simulink model "dvig"  (R2021b)
settings: Solver=ode14x  StartTime=0.0  StopTime=16  FixedStep=0.001  RelTol=1e-3
values from neighbouring files (symbols this model uses):
  F_s = 0.004    [init.m]
  Hu = 42.915e6    (= 42915000)    [init.m]
  I = 8.8e-4    (= 0.00088)    [init.m]
  i_g_arr = [377.41 480.99 586.62 694.69 805.34 918.56 1034.1 1151.8].*1000    [init.m]
  i_k_arr = [222.97 273.05 323.23 373.55 424.14 475.09 524.39 578.43].*1000    [init.m]
  K_arr = [0 1.48 2.96 4.44 5.92 7.40 8.88 10.36 11.84 13.32 14.80 22.20]    [init.m]
  k_tr_arr = [0.0174 0.087]    [init.m]
  k_v = 1.4    [init.m]
  kpd_gor = 0.98    [init.m]
  L0 = 14.627    [init.m]
  n_arr = [0 90457]    [init.m]
  R_arr = [510.7 463.9 424.2 390.9 363.4 341.2 323.5 310.9 301.3 294.0 289.6 288.2]    [init.m]
  R_v = 287    [init.m]
  sig_g = 0.955    [init.m]
  sig_s = 0.95    [init.m]
  sig_vh = 0.99    [init.m]
  T_g_arr = [373 473 573 673 773 873 973 1073]    [init.m]
  T_k_arr = [223.15 273.15 323.15 373.15 423.15 473.15 523.15 573.15]    [init.m]
  V_ks = F_ks*l_ks    (= 0.00176714586764)    [init.m]
undefined symbols (not defined in the file or in its folder): sigbuilder_block
libraries: aerolibatmos2 x1
settings Model: Creator=Admin  LastModifiedBy=admin
settings SolverCC: AlgebraicLoopSolver=TrustRegion
settings DataIOCC: ReturnWorkspaceOutputs=off
settings DebuggingCC: SFMachineParentedDataDiag=warning  ArithmeticOperatorsInVariantConditions=warning
settings SFSimCC: SimUseLocalCustomCode=off  CustomCodeUndefinedFunction=UseInterfaceOnly
settings RTWCC: RTWUseLocalCustomCode=off

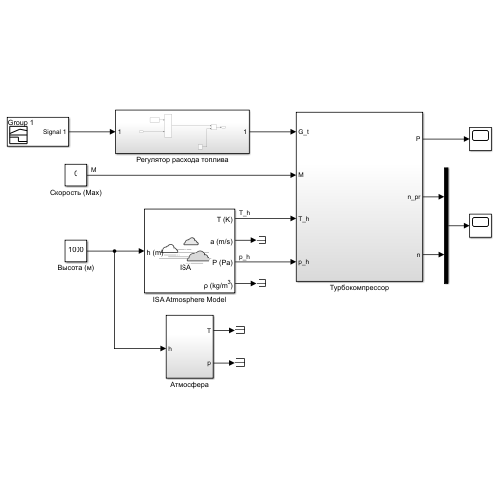
[thumbnail: Simulink's stored preview of the top-level diagram]
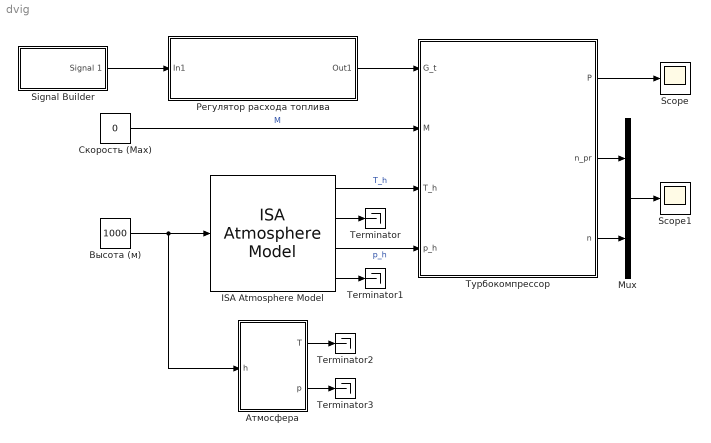
== system dvig ==
  ISA Atmosphere Model : aerolibatmos2/ISA Atmosphere Model  custom=off  g=9.80665  gamma=1.4  R=287.0531  L=0.0065  h_trop=11000  h_strat=20000  rho0=1.225  P0=101325  T0=288.15  h0=0
  Mux : Mux  Inputs=2
  Scope : Scope
  Scope1 : Scope
  Signal Builder : Subsystem  Tag=STV Subsys  LoadFcn=sigbuilder_block('load');  StartFcn=sigbuilder_block('start');  StopFcn=sigbuilder_block('stop');  ClipboardFcn=sigbuilder_block('clipboard');  mask(Sigbuilder block){tuvar=[0:10]}
      mask help: Simulink:masks:SigbuilderBlock_MD
      mask init:
      | if ~strcmp(get_param(bdroot(gcbh),'SimulationStatus'),'stopped') tuvar = sigbuilder_block('maskInit'); end
      settings: CopyFcn=sigbuilder_block('copy');  DeleteFcn=sigbuilder_block('delete');  ModelCloseFcn=sigbuilder_block('modelClose');  PreSaveFcn=sigbuilder_block('preSave');  PauseFcn=sigbuilder_block('pause');  ContinueFcn=sigbuilder_block('continue');  NameChangeFcn=sigbuilder_block('namechange');  OpenFcn=sigbuilder_block('open',[5.4 36 1141.2 516.6 ]);  CloseFcn=sigbuilder_block('close');
      mask Display: plot(0, 0, 100, 100,[2, 2, 32, 32, 2], [68, 8, 8, 68, 68],[32, 2], [38, 38], [32, 19, 2],[53, 60, 44], [32, 17, 17, 2],[16, 16, 31, 31]);txt = getActiveGroup(gcbh);text(2, 100, txt,'verticalAlignment', 'top');
  Terminator{,1..3} (4 alike) : Terminator
  Атмосфера : Subsystem
  Высота (м) : Constant  Value=1000
  Регулятор расхода топлива : Subsystem
  Скорость (Мах) : Constant  Value=0
  Турбокомпрессор : Subsystem
  wires:
  Высота (м)/1 -> Атмосфера/1(h), ISA Atmosphere Model/1
  ISA Atmosphere Model/4 -> Terminator1/1
  ISA Atmosphere Model/2 -> Terminator/1
  Скорость (Мах)/1 -> Турбокомпрессор/2(M)  "M"
  ISA Atmosphere Model/1 -> Турбокомпрессор/3(T_h)  "T_h"
  ISA Atmosphere Model/3 -> Турбокомпрессор/4(p_h)  "p_h"
  Турбокомпрессор/1(P) -> Scope/1
  Атмосфера/1(T) -> Terminator2/1
  Атмосфера/2(p) -> Terminator3/1
  Mux/1 -> Scope1/1
  Турбокомпрессор/3(n) -> Mux/2
  Турбокомпрессор/2(n_pr) -> Mux/1
  Signal Builder/1(Signal 1) -> Регулятор расхода топлива/1(In1)
  Регулятор расхода топлива/1(Out1) -> Турбокомпрессор/1(G_t)

== system dvig/Signal Builder ==
  Demux : Demux  Tag=STV Demux  Outputs=1
      settings: DisplayOption=none
  FromWs : FromWorkspace  Tag=STV FromWs  VariableName=tuvar
      SigBuilderData=|
      | common.afterFinalStr = 'Extrapolate'
      | common.sampleTime = 0
      | dataSet.timeRange = [0 16]
      | dataSet.name = 'Group 1'
      | sbobj.Groups.Name = 'Group 1'
      | sbobj.Groups.Signals.Name = 'Signal 1'
      | sbobj.Groups.Signals.XData = [0 1.06 3.8 5 6 8 10 12 14 16]
      | sbobj.Groups.Signals.YData = [0.001 0.00101 0.0023 0.0023 0.0051 0.0045 0.0078 0.0056 0.01225 0.01225]
      | sbobj.Groups.TimeRange = [0 16]
  Signal 1 : Outport  Tag=STV Outport
  wires:
  Demux/1 -> Signal 1/1
  FromWs/1 -> Demux/1

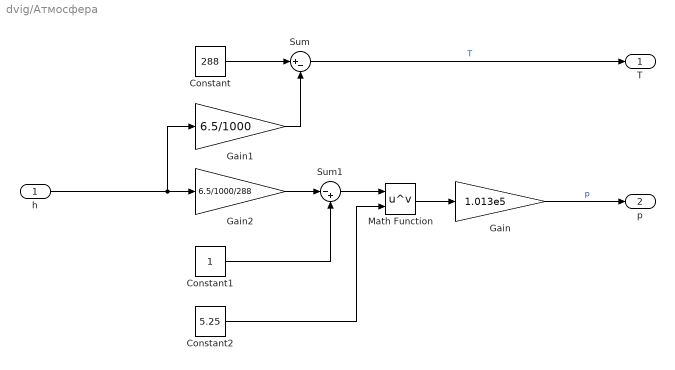
== system dvig/Атмосфера ==
  h : Inport
  Constant : Constant  Value=288
  Constant1 : Constant
  Constant2 : Constant  Value=5.25
  Gain : Gain  Gain=1.013e5
  Gain1 : Gain  Gain=6.5/1000
  Gain2 : Gain  Gain=6.5/1000/288
  Math Function : Math  Operator=pow  SaturateOnIntegerOverflow=on
  Sum : Sum  Inputs=|+-
  Sum1 : Sum  Inputs=|-+
  T : Outport  VectorParamsAs1DForOutWhenUnconnected=off
  p : Outport  Port=2  VectorParamsAs1DForOutWhenUnconnected=off
  wires:
  h/1 -> Gain1/1, Gain2/1
  Gain/1 -> p/1  "p"
  Sum1/1 -> Math Function/1
  Sum/1 -> T/1  "T"
  Constant1/1 -> Sum1/2
  Gain1/1 -> Sum/2
  Gain2/1 -> Sum1/1
  Constant2/1 -> Math Function/2
  Constant/1 -> Sum/1
  Math Function/1 -> Gain/1

== system dvig/Регулятор расхода топлива ==
  In1 : Inport
  Constant : Constant  Value=0.001
  Min : MinMax  Inputs=2
  Min1 : MinMax  Function=max  Inputs=2
  n_max : Constant  Value=0.0084
  Out1 : Outport
  wires:
  Min/1 -> Min1/1
  n_max/1 -> Min/1
  Constant/1 -> Min1/2
  Min1/1 -> Out1/1
  In1/1 -> Min/2

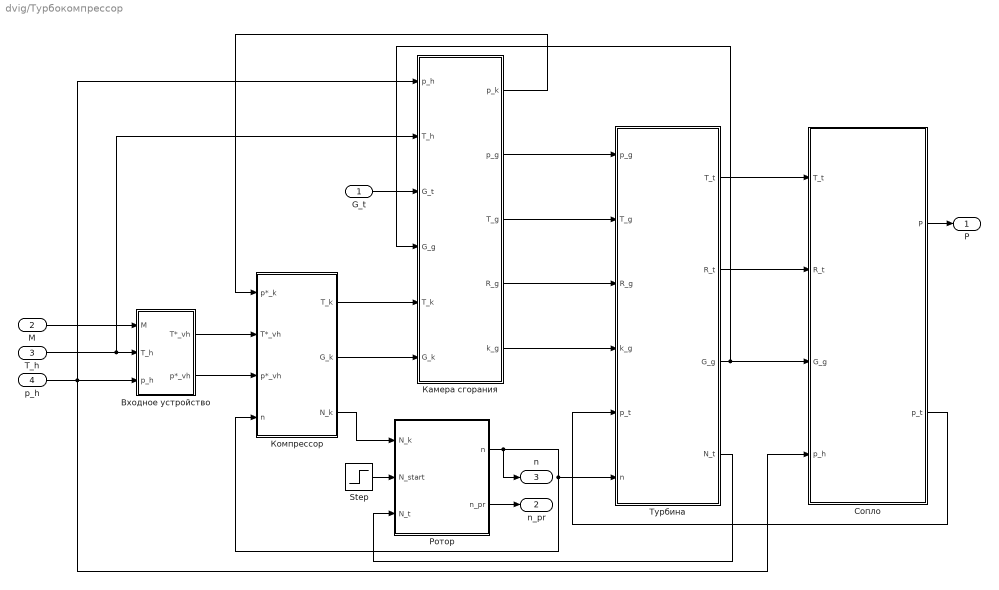
== system dvig/Турбокомпрессор ==
  G_t : Inport
  M : Inport  Port=2
  T_h : Inport  Port=3
  p_h : Inport  Port=4
  Step : Step  Time=3  Before=60000  After=0  SampleTime=0
  Входное устройство : Subsystem
  Камера сгорания : Subsystem
  Компрессор : Subsystem
  Ротор : Subsystem
  Сопло : Subsystem
  Турбина : Subsystem
  P : Outport  VectorParamsAs1DForOutWhenUnconnected=off
  n_pr : Outport  Port=2  VectorParamsAs1DForOutWhenUnconnected=off
  n : Outport  Port=3  VectorParamsAs1DForOutWhenUnconnected=off
  wires:
  G_t/1 -> Камера сгорания/3(G_t)
  Камера сгорания/1(p_k) -> Компрессор/1(p*_k)
  Входное устройство/1(T*_vh) -> Компрессор/2(T*_vh)
  Компрессор/1(T_k) -> Камера сгорания/5(T_k)
  T_h/1 -> Камера сгорания/2(T_h), Входное устройство/2(T_h)
  p_h/1 -> Камера сгорания/1(p_h), Входное устройство/3(p_h), Сопло/4(p_h)
  M/1 -> Входное устройство/1(M)
  Компрессор/2(G_k) -> Камера сгорания/6(G_k)
  Входное устройство/2(p*_vh) -> Компрессор/3(p*_vh)
  Камера сгорания/3(T_g) -> Турбина/2(T_g)
  Камера сгорания/4(R_g) -> Турбина/3(R_g)
  Камера сгорания/5(k_g) -> Турбина/4(k_g)
  Камера сгорания/2(p_g) -> Турбина/1(p_g)
  Ротор/1(n) -> n/1, Турбина/6(n), Компрессор/4(n)
  Сопло/2(p_t) -> Турбина/5(p_t)
  Компрессор/3(N_k) -> Ротор/1(N_k)
  Турбина/1(T_t) -> Сопло/1(T_t)
  Турбина/2(R_t) -> Сопло/2(R_t)
  Сопло/1(P) -> P/1
  Турбина/4(N_t) -> Ротор/3(N_t)
  Step/1 -> Ротор/2(N_start)
  Турбина/3(G_g) -> Сопло/3(G_g), Камера сгорания/4(G_g)
  Ротор/2(n_pr) -> n_pr/1

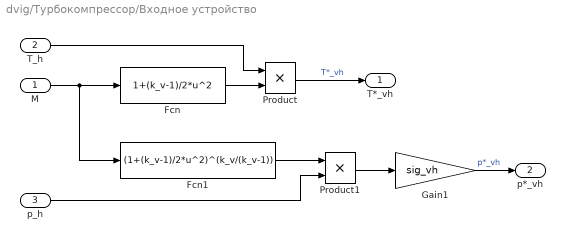
== system dvig/Турбокомпрессор/Входное устройство ==
  M : Inport
  T_h : Inport  Port=2
  p_h : Inport  Port=3
  Fcn : Fcn  Expr=1+(k_v-1)/2*u^2
  Fcn1 : Fcn  Expr=(1+(k_v-1)/2*u^2)^(k_v/(k_v-1))
  Gain1 : Gain  Gain=sig_vh
  Product : Product
  Product1 : Product
  T*_vh : Outport  VectorParamsAs1DForOutWhenUnconnected=off
  p*_vh : Outport  Port=2  VectorParamsAs1DForOutWhenUnconnected=off
  wires:
  p_h/1 -> Product1/2
  T_h/1 -> Product/1
  Product/1 -> T*_vh/1  "T*_vh"
  Fcn1/1 -> Product1/1
  Fcn/1 -> Product/2
  Gain1/1 -> p*_vh/1  "p*_vh"
  M/1 -> Fcn1/1, Fcn/1
  Product1/1 -> Gain1/1

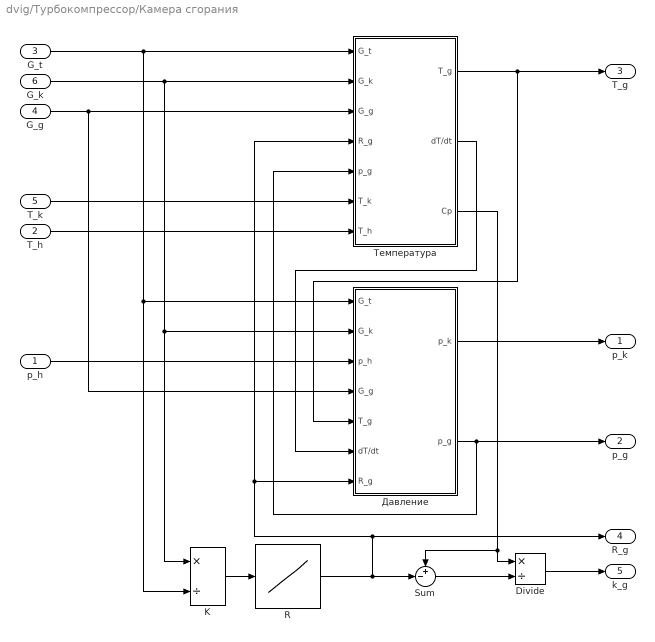
== system dvig/Турбокомпрессор/Камера сгорания ==
  p_h : Inport
  T_h : Inport  Port=2
  G_t : Inport  Port=3
  G_g : Inport  Port=4
  T_k : Inport  Port=5
  G_k : Inport  Port=6
  Divide : Product  Inputs=*/
  K : Product  Inputs=*/
  R : Lookup_n-D  NumberOfTableDimensions=1  BreakpointsForDimension1=K_arr  Table=R_arr  InternalRulePriority=Speed  RndMeth=Simplest  InputSameDT=on
  Sum : Sum  Inputs=+-|
  Давление : Subsystem
  Температура : Subsystem
  p_k : Outport  VectorParamsAs1DForOutWhenUnconnected=off
  p_g : Outport  Port=2  VectorParamsAs1DForOutWhenUnconnected=off
  T_g : Outport  Port=3  VectorParamsAs1DForOutWhenUnconnected=off
  R_g : Outport  Port=4  VectorParamsAs1DForOutWhenUnconnected=off
  k_g : Outport  Port=5  VectorParamsAs1DForOutWhenUnconnected=off
  wires:
  G_t/1 -> K/2, Давление/1(G_t), Температура/1(G_t)
  G_k/1 -> K/1, Давление/2(G_k), Температура/2(G_k)
  p_h/1 -> Давление/3(p_h)
  G_g/1 -> Давление/4(G_g), Температура/3(G_g)
  K/1 -> R/1
  R/1 -> R_g/1, Температура/4(R_g), Давление/7(R_g), Sum/2
  Sum/1 -> Divide/2
  Температура/3(Cp) -> Divide/1, Sum/1
  Давление/1(p_k) -> p_k/1
  Давление/2(p_g) -> Температура/5(p_g), p_g/1
  Температура/1(T_g) -> Давление/5(T_g), T_g/1
  Температура/2(dT/dt) -> Давление/6(dT/dt)
  T_k/1 -> Температура/6(T_k)
  T_h/1 -> Температура/7(T_h)
  Divide/1 -> k_g/1

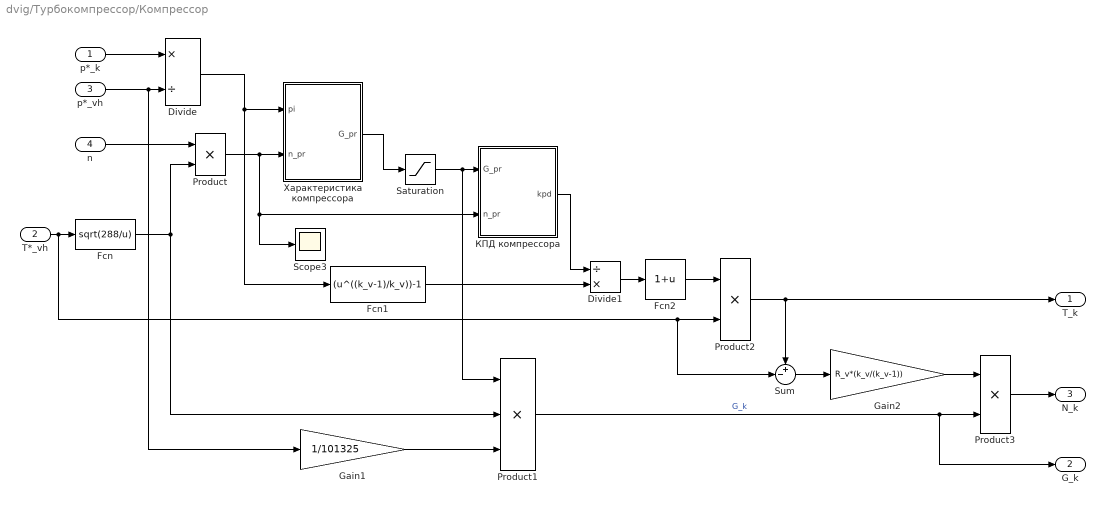
== system dvig/Турбокомпрессор/Компрессор ==
  p*_k : Inport
  T*_vh : Inport  Port=2
  p*_vh : Inport  Port=3
  n : Inport  Port=4
  Divide : Product  Inputs=*/
  Divide1 : Product  Inputs=/*
  Fcn : Fcn  Expr=sqrt(288/u)
  Fcn1 : Fcn  Expr=(u^((k_v-1)/k_v))-1
  Fcn2 : Fcn  Expr=1+u
  Gain1 : Gain  Gain=1/101325
  Gain2 : Gain  Gain=R_v*(k_v/(k_v-1))
  Product : Product
  Product1 : Product  Inputs=3
  Product2 : Product
  Product3 : Product
  Saturation : Saturate  UpperLimit=0.8  LowerLimit=0.05
  Scope3 : Scope
  Sum : Sum  Inputs=+-|
  КПД компрессора : MATLAB Function  TreatAsAtomicUnit=on
  Характеристика компрессора : MATLAB Function  TreatAsAtomicUnit=on
  T_k : Outport  VectorParamsAs1DForOutWhenUnconnected=off
  G_k : Outport  Port=2  VectorParamsAs1DForOutWhenUnconnected=off
  N_k : Outport  Port=3  VectorParamsAs1DForOutWhenUnconnected=off
  wires:
  p*_k/1 -> Divide/1
  Divide/1 -> Fcn1/1, Характеристика компрессора/1(pi)
  Saturation/1 -> Product1/1, КПД компрессора/1(G_pr)
  p*_vh/1 -> Gain1/1, Divide/2
  Fcn2/1 -> Product2/1
  Gain1/1 -> Product1/3
  Fcn/1 -> Product1/2, Product/2
  Divide1/1 -> Fcn2/1
  Sum/1 -> Gain2/1
  Product/1 -> Scope3/1, КПД компрессора/2(n_pr), Характеристика компрессора/2(n_pr)
  n/1 -> Product/1
  Gain2/1 -> Product3/1
  Product1/1 -> G_k/1, Product3/2  "G_k"
  Product3/1 -> N_k/1
  T*_vh/1 -> Sum/2, Product2/2, Fcn/1
  КПД компрессора/1(kpd) -> Divide1/1
  Product2/1 -> T_k/1, Sum/1
  Fcn1/1 -> Divide1/2
  Характеристика компрессора/1(G_pr) -> Saturation/1

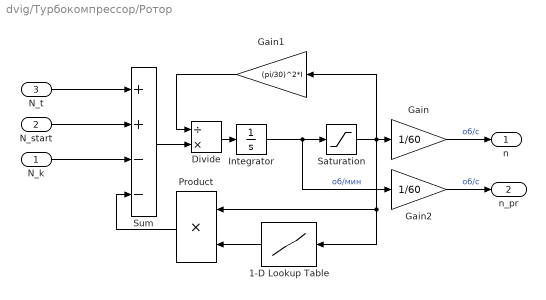
== system dvig/Турбокомпрессор/Ротор ==
  N_k : Inport
  N_start : Inport  Port=2
  N_t : Inport  Port=3
  1-D Lookup Table : Lookup_n-D  NumberOfTableDimensions=1  BreakpointsForDimension1=n_arr  Table=k_tr_arr  InternalRulePriority=Speed  RndMeth=Simplest  InputSameDT=on
  Divide : Product  Inputs=/*
  Gain : Gain  Gain=1/60
  Gain1 : Gain  Gain=(pi/30)^2*I
  Gain2 : Gain  Gain=1/60
  Integrator : Integrator
  Product : Product
  Saturation : Saturate  UpperLimit=90500  LowerLimit=1
  Sum : Sum  Inputs=++--
  n : Outport  VectorParamsAs1DForOutWhenUnconnected=off
  n_pr : Outport  Port=2  VectorParamsAs1DForOutWhenUnconnected=off
  wires:
  N_k/1 -> Sum/3
  N_t/1 -> Sum/1
  Saturation/1 -> 1-D Lookup Table/1, Product/1, Gain/1, Gain1/1
  Integrator/1 -> Gain2/1, Saturation/1  "об/мин"
  Gain/1 -> n/1  "об/с"
  Sum/1 -> Divide/2
  Divide/1 -> Integrator/1
  Gain1/1 -> Divide/1
  1-D Lookup Table/1 -> Product/2
  Product/1 -> Sum/4
  N_start/1 -> Sum/2
  Gain2/1 -> n_pr/1  "об/с"

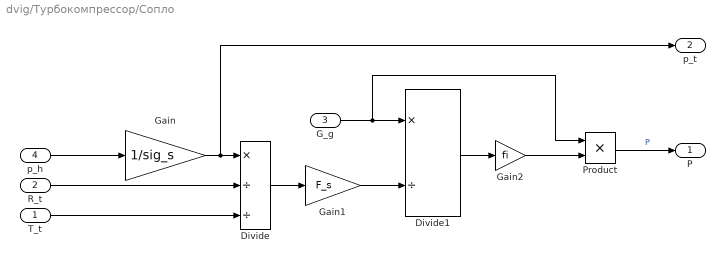
== system dvig/Турбокомпрессор/Сопло ==
  T_t : Inport
  R_t : Inport  Port=2
  G_g : Inport  Port=3
  p_h : Inport  Port=4
  Divide : Product  Inputs=*//
  Divide1 : Product  Inputs=*/
  Gain : Gain  Gain=1/sig_s
  Gain1 : Gain  Gain=F_s
  Gain2 : Gain  Gain=fi
  Product : Product
  P : Outport  VectorParamsAs1DForOutWhenUnconnected=off
  p_t : Outport  Port=2  VectorParamsAs1DForOutWhenUnconnected=off
  wires:
  T_t/1 -> Divide/3
  p_h/1 -> Gain/1
  R_t/1 -> Divide/2
  Divide1/1 -> Gain2/1
  G_g/1 -> Product/1, Divide1/1
  Product/1 -> P/1  "P"
  Divide/1 -> Gain1/1
  Gain2/1 -> Product/2
  Gain/1 -> p_t/1, Divide/1
  Gain1/1 -> Divide1/2

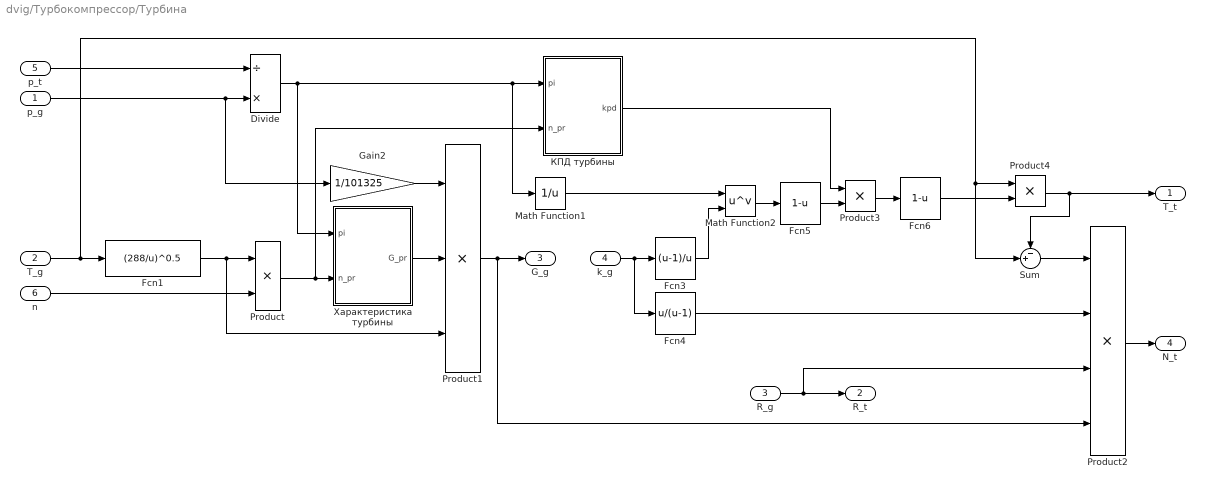
== system dvig/Турбокомпрессор/Турбина ==
  p_g : Inport
  T_g : Inport  Port=2
  R_g : Inport  Port=3
  k_g : Inport  Port=4
  p_t : Inport  Port=5
  n : Inport  Port=6
  Divide : Product  Inputs=/*
  Fcn1 : Fcn  Expr=(288/u)^0.5
  Fcn3 : Fcn  Expr=(u-1)/u
  Fcn4 : Fcn  Expr=u/(u-1)
  Fcn5 : Fcn  Expr=1-u
  Fcn6 : Fcn  Expr=1-u
  Gain2 : Gain  Gain=1/101325
  Math Function1 : Math  Operator=reciprocal  SignedPower=on  SaturateOnIntegerOverflow=on
  Math Function2 : Math  Operator=pow  SaturateOnIntegerOverflow=on
  Product : Product
  Product1 : Product  Inputs=3
  Product2 : Product  Inputs=4
  Product3 : Product
  Product4 : Product
  Sum : Sum  Inputs=-+|
  КПД турбины : MATLAB Function  TreatAsAtomicUnit=on
  Характеристика турбины : MATLAB Function  TreatAsAtomicUnit=on
  T_t : Outport  VectorParamsAs1DForOutWhenUnconnected=off
  R_t : Outport  Port=2  VectorParamsAs1DForOutWhenUnconnected=off
  G_g : Outport  Port=3  VectorParamsAs1DForOutWhenUnconnected=off
  N_t : Outport  Port=4  VectorParamsAs1DForOutWhenUnconnected=off
  wires:
  n/1 -> Product/2
  p_t/1 -> Divide/1
  p_g/1 -> Gain2/1, Divide/2
  Divide/1 -> Math Function1/1, КПД турбины/1(pi), Характеристика турбины/1(pi)
  Fcn1/1 -> Product1/3, Product/1
  R_g/1 -> Product2/3, R_t/1
  Product/1 -> КПД турбины/2(n_pr), Характеристика турбины/2(n_pr)
  Product1/1 -> G_g/1, Product2/4
  Fcn3/1 -> Math Function2/2
  k_g/1 -> Fcn4/1, Fcn3/1
  Fcn4/1 -> Product2/2
  Math Function2/1 -> Fcn5/1
  Fcn5/1 -> Product3/2
  Product3/1 -> Fcn6/1
  Product2/1 -> N_t/1
  Fcn6/1 -> Product4/2
  Product4/1 -> Sum/1, T_t/1
  Sum/1 -> Product2/1
  T_g/1 -> Sum/2, Product4/1, Fcn1/1
  Math Function1/1 -> Math Function2/1
  Характеристика турбины/1(G_pr) -> Product1/2
  КПД турбины/1(kpd) -> Product3/1
  Gain2/1 -> Product1/1

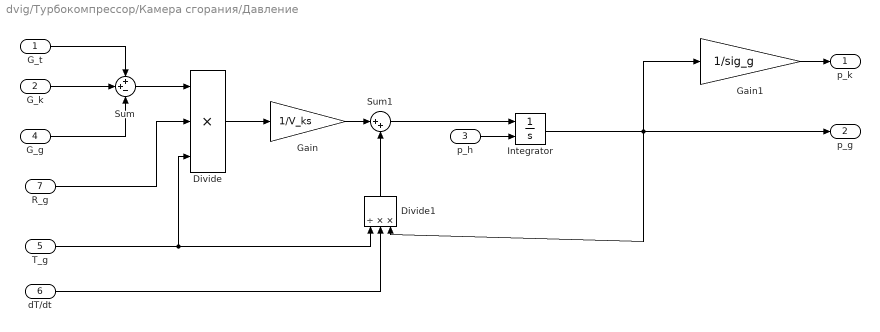
== system dvig/Турбокомпрессор/Камера сгорания/Давление ==
  G_t : Inport
  G_k : Inport  Port=2
  p_h : Inport  Port=3
  G_g : Inport  Port=4
  T_g : Inport  Port=5
  dT/dt : Inport  Port=6
  R_g : Inport  Port=7
  Divide : Product  Inputs=3
  Divide1 : Product  Inputs=/**
  Gain : Gain  Gain=1/V_ks
  Gain1 : Gain  Gain=1/sig_g
  Integrator : Integrator  InitialConditionSource=external
  Sum : Sum  Inputs=++-
  Sum1 : Sum  Inputs=|++
  p_k : Outport  VectorParamsAs1DForOutWhenUnconnected=off
  p_g : Outport  Port=2  VectorParamsAs1DForOutWhenUnconnected=off
  wires:
  Gain1/1 -> p_k/1
  Integrator/1 -> Divide1/3, p_g/1, Gain1/1
  G_g/1 -> Sum/3
  G_k/1 -> Sum/2
  G_t/1 -> Sum/1
  Gain/1 -> Sum1/1
  Divide/1 -> Gain/1
  Sum/1 -> Divide/1
  T_g/1 -> Divide1/1, Divide/3
  p_h/1 -> Integrator/2
  Divide1/1 -> Sum1/2
  Sum1/1 -> Integrator/1
  dT/dt/1 -> Divide1/2
  R_g/1 -> Divide/2

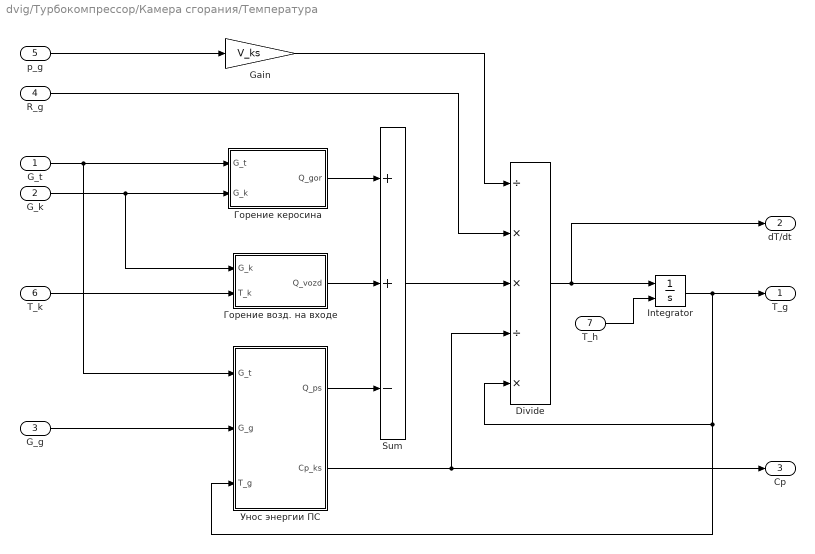
== system dvig/Турбокомпрессор/Камера сгорания/Температура ==
  G_t : Inport
  G_k : Inport  Port=2
  G_g : Inport  Port=3
  R_g : Inport  Port=4
  p_g : Inport  Port=5
  T_k : Inport  Port=6
  T_h : Inport  Port=7
  Divide : Product  Inputs=/**/*
  Gain : Gain  Gain=V_ks
  Integrator : Integrator  InitialConditionSource=external
  Sum : Sum  Inputs=++-
  Горение возд. на входе : Subsystem
  Горение керосина : Subsystem
  Унос энергии ПС : Subsystem
  T_g : Outport  VectorParamsAs1DForOutWhenUnconnected=off
  dT/dt : Outport  Port=2  VectorParamsAs1DForOutWhenUnconnected=off
  Cp : Outport  Port=3  VectorParamsAs1DForOutWhenUnconnected=off
  wires:
  G_t/1 -> Унос энергии ПС/1(G_t), Горение керосина/1(G_t)
  G_k/1 -> Горение возд. на входе/1(G_k), Горение керосина/2(G_k)
  Горение керосина/1(Q_gor) -> Sum/1
  Sum/1 -> Divide/3
  R_g/1 -> Divide/2
  p_g/1 -> Gain/1
  Gain/1 -> Divide/1
  T_h/1 -> Integrator/2
  Divide/1 -> Integrator/1, dT/dt/1
  Integrator/1 -> T_g/1, Унос энергии ПС/3(T_g), Divide/5
  T_k/1 -> Горение возд. на входе/2(T_k)
  Горение возд. на входе/1(Q_vozd) -> Sum/2
  G_g/1 -> Унос энергии ПС/2(G_g)
  Унос энергии ПС/1(Q_ps) -> Sum/3
  Унос энергии ПС/2(Cp_ks) -> Cp/1, Divide/4

== system dvig/Турбокомпрессор/Камера сгорания/Температура/Горение возд. на входе ==
  G_k : Inport
  T_k : Inport  Port=2
  Divide1 : Product  Inputs=*/
  Product : Product  Inputs=3
  i_k : Lookup_n-D  NumberOfTableDimensions=1  BreakpointsForDimension1=T_k_arr  Table=i_k_arr  InternalRulePriority=Speed  RndMeth=Simplest  InputSameDT=on
  Q_vozd : Outport  VectorParamsAs1DForOutWhenUnconnected=off
  wires:
  Product/1 -> Q_vozd/1
  G_k/1 -> Product/1
  Divide1/1 -> Product/2
  i_k/1 -> Divide1/1
  T_k/1 -> Divide1/2, Product/3, i_k/1

== system dvig/Турбокомпрессор/Камера сгорания/Температура/Горение керосина ==
  G_t : Inport
  G_k : Inport  Port=2
  Gain : Gain  Gain=1/L0
  Gain1 : Gain  Gain=Hu*kpd_gor
  MinMax : MinMax  Inputs=2
  Q_gor : Outport  VectorParamsAs1DForOutWhenUnconnected=off
  wires:
  MinMax/1 -> Gain1/1
  G_t/1 -> MinMax/1
  G_k/1 -> Gain/1
  Gain1/1 -> Q_gor/1  "Q_gor"
  Gain/1 -> MinMax/2

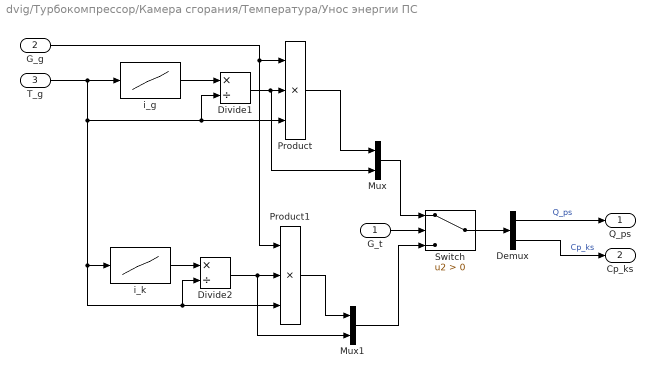
== system dvig/Турбокомпрессор/Камера сгорания/Температура/Унос энергии ПС ==
  G_t : Inport
  G_g : Inport  Port=2
  T_g : Inport  Port=3
  Demux : Demux  Outputs=2
  Divide1 : Product  Inputs=*/
  Divide2 : Product  Inputs=*/
  Mux : Mux  Inputs=2
  Mux1 : Mux  Inputs=2
  Product : Product  Inputs=3
  Product1 : Product  Inputs=3
  Switch : Switch  Criteria=u2 > Threshold
  i_g : Lookup_n-D  NumberOfTableDimensions=1  BreakpointsForDimension1=T_g_arr  Table=i_g_arr  InternalRulePriority=Speed  RndMeth=Simplest  InputSameDT=on
  i_k : Lookup_n-D  NumberOfTableDimensions=1  BreakpointsForDimension1=T_k_arr  Table=i_k_arr  InternalRulePriority=Speed  RndMeth=Simplest  InputSameDT=on
  Q_ps : Outport  VectorParamsAs1DForOutWhenUnconnected=off
  Cp_ks : Outport  Port=2  VectorParamsAs1DForOutWhenUnconnected=off
  wires:
  Divide2/1 -> Mux1/2, Product1/2
  G_t/1 -> Switch/2
  Demux/2 -> Cp_ks/1  "Cp_ks"
  Mux1/1 -> Switch/3
  i_k/1 -> Divide2/1
  Product1/1 -> Mux1/1
  Mux/1 -> Switch/1
  i_g/1 -> Divide1/1
  Demux/1 -> Q_ps/1  "Q_ps"
  Switch/1 -> Demux/1
  Divide1/1 -> Mux/2, Product/2
  G_g/1 -> Product1/1, Product/1
  Product/1 -> Mux/1
  T_g/1 -> Divide2/2, Product1/3, i_k/1, Divide1/2, Product/3, i_g/1

== matlab function dvig/Турбокомпрессор/Турбина/Характеристика турбины ==
  data: pi input; n_pr input; G_pr output
%function G_pr = inter(pi,n_pr)
function G_pr = inter(pi, n_pr)
    mas = [0 381.82 534.53 686.8 763.6 836.5 ...
    1 1.0000 1.0000 1.0000 1.0000 1.0000 ...
    1 1.2000 1.2000 1.2000 1.2000 1.2000 ...
    1 1.5500 1.5328 1.5321 1.5316 1.5327 ...
    1 1.7000 1.7300 1.7418 1.7413 1.7409 ...
    1 2.0216 2.0172 2.0170 2.0169 2.0168 ...
    1 3.4511 3.4473 3.4496 3.4509 3.4509 ...
    1 4.7626 4.7530 4.7589 4.7605 4.8437 ...
    1 6.1721 6.2159 6.3032 6.3527 6.3440 ...
    0 0.000000 0.000000 0.000000 0.000000 0.000000 ...
    0 0.220000 0.225000 0.220000 0.215000 0.216000 ...
    0 0.292801 0.296743 0.297500 0.297700 0.298700 ...
    0 0.303760 0.306989 0.309100 0.309585 0.310585 ...
    0 0.311119 0.315387 0.316097 0.316300 0.317300 ...
    0 0.318322 0.320272 0.320966 0.321209 0.322209 ...
    0 0.318560 0.320411 0.321058 0.321212 0.322212 ...
    0 0.318617 0.320429 0.321185 0.321266 0.322266];

    M = 16;
    N = 6;

    N1 = M/2;
    Gkpd = zeros(1,M);
    k1 = 0;
    k2 = 0;
    XA = 0;
    XB = 0;
    kpd = 0;
    
    %
    G_pr = 0;
    %
    if n_pr>mas(N)
        kp=1+N-2;
        ks=1+N-1;
        XA=mas(kp);
        XB=mas(ks);
        k1=1-2+N*2;
        k2=1-1+N*2;

        for i=1:1:M
            kq=k1+(i-1)*N;
            kw=k2+(i-1)*N;
            if XB==XA
                XB=XB+0.1;
            end

            Gkpd(i)=mas(kq)+(((mas(kw)-mas(kq))*(n_pr-XA))/(XB-XA));
        end

    end
    
    if n_pr<mas(1)
        XA=mas(1);
        XB=mas(2);
        k1=N+1;
        k2=N+2;
        for i=1:1:M
            kq=k1+(i-1)*N;
            kw=k2+(i-1)*N;
            if XB==XA
                XB=XB+0.1;
            end
    
            Gkpd(i)=mas(kq)+(((mas(kw)-mas(kq))*(n_pr-XA))/(XB-XA));
        end
    
    else
        for i=1:1:N-1
            if n_pr>=mas(i)
                if n_pr<=mas(i+1)
                    XA=mas(i);
                    XB=mas(i+1);
                    k1=N+i;
                    k2=1+N+i;
                else
                    continue;
                end
            end
        end
    
        for i1=1:1:M
            kq=k1+(i1-1)*N;
            kw=k2+(i1-1)*N;
            if XB==XA
                XB=XB+0.1;
            end
        
            Gkpd(i1)=mas(kq)+(((mas(kw)-mas(kq))*(n_pr-XA))/(XB-XA));
        end
    end
    
    if pi>Gkpd(N1)
        kp=1+N1-2;
        ks=1+N1-1;
        XA=Gkpd(kp);
        XB=Gkpd(ks);
        k1=1-2+N1*2;
        k2=1-1+N1*2;
        kq=k1;
        kw=k2;
        if XB==XA
            XB=XB+0.1;
        end
        G_pr=Gkpd(kq)+(((Gkpd(kw)-Gkpd(kq))*(pi-XA))/(XB-XA));
    end
    if pi<Gkpd(1)
        XA=Gkpd(1);
        XB=Gkpd(2);
        k1=N1+1;
        k2=N1+2;
        kq=k1;
        kw=k2;
        if XB==XA
            XB=XB+0.1;
        end
        G_pr=Gkpd(kq)+(((Gkpd(kw)-Gkpd(kq))*(pi-XA))/(XB-XA));
        else
            for i=1:1:N1-1
                if pi>=Gkpd(i)
                    if pi<=Gkpd(i+1)
                        XA=Gkpd(i);
                        XB=Gkpd(i+1);
                        k1=N1+i;
                        k2=1+N1+i;
                    else
                        continue;
                    end
    
                end
    
                kq=k1;
                kw=k2;
                if XB==XA
                    XB=XB+0.1;
                end
                G_pr=Gkpd(kq)+(((Gkpd(kw)-Gkpd(kq))*(pi-XA))/(XB-XA));
            end
    end  
end

== matlab function dvig/Турбокомпрессор/Компрессор/КПД компрессора ==
  data: G_pr input; kpd output; n_pr input
function kpd = inter(G_pr,n_pr)
    mas = [568.67 853 995.78 1138 1279.5 1422.6 1558.3 ...
    0.0000 0.0000 0.0000 0.0000 0.0000 0.0000 0.0000 ...
    0.1977 0.3376 0.3112 0.4679 0.5079 0.6247 0.6913 ...
    0.2613 0.4048 0.4290 0.5524 0.6464 0.7283 0.7787 ...
    0.2918 0.4196 0.5063 0.5899 0.6758 0.7469 0.7915 ...
    0.3200 0.4328 0.5070 0.5900 0.6770 0.7490 0.7920 ...
    0.5000 0.5000 0.5000 0.5000 0.5000 0.5000 0.5000 ...
    0.7500 0.8264 0.7700 0.7946 0.7655 0.7515 0.7241 ...
    0.8289 0.7396 0.8218 0.7963 0.7846 0.7491 0.7191 ...
    0.7069 0.6439 0.5610 0.6148 0.6969 0.6977 0.6228 ...
    0.4000 0.4000 0.4000 0.4000 0.4000 0.4000 0.4000];
    M = 10;
    N = 7;
    
    N1 = M/2;
    Gkpd = zeros(1,M);
    k1 = 0;
    k2 = 0;
    XA = 0;
    XB = 0;
    kpd = 0;
    
    if n_pr>mas(N)
        kp=1+N-2;
        ks=1+N-1;
        XA=mas(kp);
        XB=mas(ks);
        k1=1-2+N*2;
        k2=1-1+N*2;

        for i=1:1:M
            kq=k1+(i-1)*N;
            kw=k2+(i-1)*N;
            if XB==XA
                XB=XB+0.1;
            end

            Gkpd(i)=mas(kq)+(((mas(kw)-mas(kq))*(n_pr-XA))/(XB-XA));
        end

    end
    
    if n_pr<mas(1)
        XA=mas(1);
        XB=mas(2);
        k1=N+1;
        k2=N+2;
        for i=1:1:M
            kq=k1+(i-1)*N;
            kw=k2+(i-1)*N;
            if XB==XA
                XB=XB+0.1;
            end
    
            Gkpd(i)=mas(kq)+(((mas(kw)-mas(kq))*(n_pr-XA))/(XB-XA));
        end
    
    else
        for i=1:1:N-1
            if n_pr>=mas(i)
                if n_pr<=mas(i+1)
                    XA=mas(i);
                    XB=mas(i+1);
                    k1=N+i;
                    k2=1+N+i;
                else
                    continue;
                end
            end
        end
    
        for i1=1:1:M
            kq=k1+(i1-1)*N;
            kw=k2+(i1-1)*N;
            if XB==XA
                XB=XB+0.1;
            end
        
            Gkpd(i1)=mas(kq)+(((mas(kw)-mas(kq))*(n_pr-XA))/(XB-XA));
        end
    end
    
    if G_pr>Gkpd(N1)
        kp=1+N1-2;
        ks=1+N1-1;
        XA=Gkpd(kp);
        XB=Gkpd(ks);
        k1=1-2+N1*2;
        k2=1-1+N1*2;
        kq=k1;
        kw=k2;
        if XB==XA
            XB=XB+0.1;
        end
        kpd=Gkpd(kq)+(((Gkpd(kw)-Gkpd(kq))*(G_pr-XA))/(XB-XA));
    end
    if G_pr<Gkpd(1)
        XA=Gkpd(1);
        XB=Gkpd(2);
        k1=N1+1;
        k2=N1+2;
        kq=k1;
        kw=k2;
        if XB==XA
            XB=XB+0.1;
        end
        kpd=Gkpd(kq)+(((Gkpd(kw)-Gkpd(kq))*(G_pr-XA))/(XB-XA));
        else
            for i=1:1:N1-1
                if G_pr>=Gkpd(i)
                    if G_pr<=Gkpd(i+1)
                        XA=Gkpd(i);
                        XB=Gkpd(i+1);
                        k1=N1+i;
                        k2=1+N1+i;
                    else
                        continue;
                    end
    
                end
    
                kq=k1;
                kw=k2;
                if XB==XA
                    XB=XB+0.1;
                end
                kpd=Gkpd(kq)+(((Gkpd(kw)-Gkpd(kq))*(G_pr-XA))/(XB-XA));
            end
    end  
end

== matlab function dvig/Турбокомпрессор/Компрессор/Характеристика компрессора ==
  data: pi input; n_pr input; G_pr output
function G_pr = inter(pi,n_pr)

     mas = [0 568.67 853    995.78 1138   1279.5 1422.6 1558.3 ...
            1 1.00   1.22   1.36   1.54   1.80   2.00   2.15 ...
            1 1.00   1.31   1.49   1.79   2.50   3.02   4.25 ...
            1 1.09   1.40   1.69   1.99   2.83   3.37   4.71 ...
            1 1.09   1.50   1.89   2.30   3.04   3.82   4.82 ...
            1 1.18   1.60   2.00   2.46   3.17   3.96   4.93 ...
            1 1.23   1.70   2.08   2.53   3.22   4.02   4.96 ...
            1 1.28   1.78   2.12   2.59   3.22   4.02   4.96 ...
            0 0.3200 0.4328 0.5063 0.5899 0.6770 0.7482 0.7916 ...
            0 0.3200 0.4285 0.5063 0.5898 0.6702 0.7448 0.7843 ...
            0 0.2918 0.4194 0.4956 0.5848 0.6464 0.7360 0.7542 ...
            0 0.2918 0.4049 0.4649 0.5524 0.5914 0.6792 0.7316 ...
            0 0.2613 0.3803 0.4290 0.5070 0.5265 0.6247 0.6913 ...
            0 0.2295 0.3376 0.3899 0.4679 0.4675 0.5848 0.6616 ...
            0 0.1977 0.2640 0.3112 0.3478 0.3897 0.4294 0.5072];
    M = 14;
    N = 8;

    N1 = M/2;
    Gkpd = zeros(1,M);
    k1 = 0;
    k2 = 0;
    XA = 0;
    XB = 0;
    kpd = 0;
    
    %
    G_pr = 0;
    %
    if n_pr>mas(N)
        kp=1+N-2;
        ks=1+N-1;
        XA=mas(kp);
        XB=mas(ks);
        k1=1-2+N*2;
        k2=1-1+N*2;

        for i=1:1:M
            kq=k1+(i-1)*N;
            kw=k2+(i-1)*N;
            if XB==XA
                XB=XB+0.1;
            end

            Gkpd(i)=mas(kq)+(((mas(kw)-mas(kq))*(n_pr-XA))/(XB-XA));
        end

    end
    
    if n_pr<mas(1)
        XA=mas(1);
        XB=mas(2);
        k1=N+1;
        k2=N+2;
        for i=1:1:M
            kq=k1+(i-1)*N;
            kw=k2+(i-1)*N;
            if XB==XA
                XB=XB+0.1;
            end
    
            Gkpd(i)=mas(kq)+(((mas(kw)-mas(kq))*(n_pr-XA))/(XB-XA));
        end
    
    else
        for i=1:1:N-1
            if n_pr>=mas(i)
                if n_pr<=mas(i+1)
                    XA=mas(i);
                    XB=mas(i+1);
                    k1=N+i;
                    k2=1+N+i;
                else
                    continue;
                end
            end
        end
    
        for i1=1:1:M
            kq=k1+(i1-1)*N;
            kw=k2+(i1-1)*N;
            if XB==XA
                XB=XB+0.1;
            end
        
            Gkpd(i1)=mas(kq)+(((mas(kw)-mas(kq))*(n_pr-XA))/(XB-XA));
        end
    end
    
    if pi>Gkpd(N1)
        kp=1+N1-2;
        ks=1+N1-1;
        XA=Gkpd(kp);
        XB=Gkpd(ks);
        k1=1-2+N1*2;
        k2=1-1+N1*2;
        kq=k1;
        kw=k2;
        if XB==XA
            XB=XB+0.1;
        end
        G_pr=Gkpd(kq)+(((Gkpd(kw)-Gkpd(kq))*(pi-XA))/(XB-XA));
    end
    if pi<Gkpd(1)
        XA=Gkpd(1);
        XB=Gkpd(2);
        k1=N1+1;
        k2=N1+2;
        kq=k1;
        kw=k2;
        if XB==XA
            XB=XB+0.1;
        end
        G_pr=Gkpd(kq)+(((Gkpd(kw)-Gkpd(kq))*(pi-XA))/(XB-XA));
        else
            for i=1:1:N1-1
                if pi>=Gkpd(i)
                    if pi<=Gkpd(i+1)
                        XA=Gkpd(i);
                        XB=Gkpd(i+1);
                        k1=N1+i;
                        k2=1+N1+i;
                    else
                        continue;
                    end
    
                end
    
                kq=k1;
                kw=k2;
                if XB==XA
                    XB=XB+0.1;
                end
                G_pr=Gkpd(kq)+(((Gkpd(kw)-Gkpd(kq))*(pi-XA))/(XB-XA));
            end
    end  
end

== matlab function dvig/Турбокомпрессор/Турбина/КПД турбины ==
  data: pi input; n_pr input; kpd output
function kpd = inter(pi,n_pr)
    mas = [381.82 534.53 686.8 763.6 836.5 ...
    1.0000 1.0000 1.0000 1.0000 1.0000 ...
    1.1200 1.2000 1.3000 1.5316 1.5327 ...
    1.5334 1.5328 1.6000 1.7742 1.8663 ...
    1.7000 1.7419 2.0170 2.0169 2.2000 ...
    2.0216 2.0172 2.7374 2.7373 2.8255 ...
    3.4511 3.4473 3.4496 3.4509 3.4509 ...
    4.7626 4.7530 4.7589 4.7605 4.8437 ...
    6.1721 6.2159 6.3032 6.3527 6.3440 ...
    0.5000 0.5000 0.5000 0.5000 0.5000 ...
    0.7200 0.7400 0.7400 0.7387 0.7000 ...
    0.6487 0.7440 0.7800 0.7591 0.7400 ...
    0.6100 0.7212 0.7659 0.7794 0.7800 ...
    0.5727 0.6947 0.7333 0.7596 0.7574 ...
    0.4734 0.5992 0.6849 0.7129 0.7349 ...
    0.4179 0.5305 0.6093 0.6376 0.6030 ...
    0.3758 0.4760 0.5453 0.5599 0.3884];
    
    M = 16;
    N = 5;

    N1 = M/2;
    Gkpd = zeros(1,M);
    k1 = 0;
    k2 = 0;
    XA = 0;
    XB = 0;
    kpd = 0;
 
    if n_pr>mas(N)
        kp=1+N-2;
        ks=1+N-1;
        XA=mas(kp);
        XB=mas(ks);
        k1=1-2+N*2;
        k2=1-1+N*2;

        for i=1:1:M
            kq=k1+(i-1)*N;
            kw=k2+(i-1)*N;
            if XB==XA
                XB=XB+0.1;
            end

            Gkpd(i)=mas(kq)+(((mas(kw)-mas(kq))*(n_pr-XA))/(XB-XA));
        end

    end
    
    if n_pr<mas(1)
        XA=mas(1);
        XB=mas(2);
        k1=N+1;
        k2=N+2;
        for i=1:1:M
            kq=k1+(i-1)*N;
            kw=k2+(i-1)*N;
            if XB==XA
                XB=XB+0.1;
            end
    
            Gkpd(i)=mas(kq)+(((mas(kw)-mas(kq))*(n_pr-XA))/(XB-XA));
        end
    
    else
        for i=1:1:N-1
            if n_pr>=mas(i)
                if n_pr<=mas(i+1)
                    XA=mas(i);
                    XB=mas(i+1);
                    k1=N+i;
                    k2=1+N+i;
                else
                    continue;
                end
            end
        end
    
        for i1=1:1:M
            kq=k1+(i1-1)*N;
            kw=k2+(i1-1)*N;
            if XB==XA
                XB=XB+0.1;
            end
        
            Gkpd(i1)=mas(kq)+(((mas(kw)-mas(kq))*(n_pr-XA))/(XB-XA));
        end
    end
    
    if pi>Gkpd(N1)
        kp=1+N1-2;
        ks=1+N1-1;
        XA=Gkpd(kp);
        XB=Gkpd(ks);
        k1=1-2+N1*2;
        k2=1-1+N1*2;
        kq=k1;
        kw=k2;
        if XB==XA
            XB=XB+0.1;
        end
        kpd=Gkpd(kq)+(((Gkpd(kw)-Gkpd(kq))*(pi-XA))/(XB-XA));
    end
    if pi<Gkpd(1)
        XA=Gkpd(1);
        XB=Gkpd(2);
        k1=N1+1;
        k2=N1+2;
        kq=k1;
        kw=k2;
        if XB==XA
            XB=XB+0.1;
        end
        kpd=Gkpd(kq)+(((Gkpd(kw)-Gkpd(kq))*(pi-XA))/(XB-XA));
        else
            for i=1:1:N1-1
                if pi>=Gkpd(i)
                    if pi<=Gkpd(i+1)
                        XA=Gkpd(i);
                        XB=Gkpd(i+1);
                        k1=N1+i;
                        k2=1+N1+i;
                    else
                        continue;
                    end
    
                end
    
                kq=k1;
                kw=k2;
                if XB==XA
                    XB=XB+0.1;
                end
                kpd=Gkpd(kq)+(((Gkpd(kw)-Gkpd(kq))*(pi-XA))/(XB-XA));
            end
    end  
end
